simulink model "a8_AnregungReibung_lsg"  (R2020b)
settings: Solver=ode45  StartTime=0.0  StopTime=100.0  MaxStep=0.1  RelTol=1e-3
model workspace (MAT data in the model file):
  d = 0.4
  w = 1
  w0 = 2.2360679775
settings Model: Creator=Reichl  LastModifiedBy=jakob
settings DataIOCC: ReturnWorkspaceOutputs=off
settings DebuggingCC: ArithmeticOperatorsInVariantConditions=warning
settings SFSimCC: SimUseLocalCustomCode=off  CustomCodeUndefinedFunction=UseInterfaceOnly
settings RTWCC: RTWUseLocalCustomCode=off
settings CodeAppCC: StateflowObjectComments=on

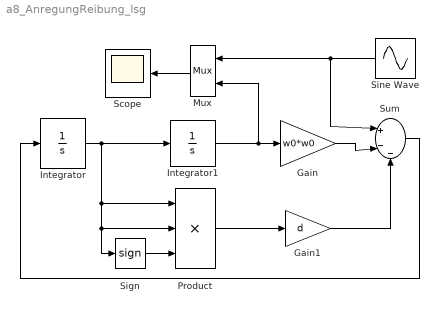
== system a8_AnregungReibung_lsg ==
  Gain : Gain  Gain=w0*w0
  Gain1 : Gain  Gain=d
  Integrator : Integrator
  Integrator1 : Integrator
  Mux : Mux  Inputs=2
  Product : Product  Inputs=3
  Scope : Scope
  Sign : Signum
  Sine Wave : Sin  Frequency=w  SampleTime=0
  Sum : Sum  Inputs=|+--
  wires:
  Sign/1 -> Product/3
  Mux/1 -> Scope/1
  Product/1 -> Gain1/1
  Integrator/1 -> Integrator1/1, Product/1, Sign/1, Product/2
  Integrator1/1 -> Mux/2, Gain/1
  Sine Wave/1 -> Mux/1, Sum/1
  Gain1/1 -> Sum/3
  Gain/1 -> Sum/2
  Sum/1 -> Integrator/1
